simulink model "TractorTrailer6DOF"  (R2023b)
settings: Solver=ode23tb  StartTime=0.0  StopTime=50  MaxStep=1.0  RelTol=1e-1  AbsTol=1e-5
model mask{initialTractorPosition=[0 0 0], initialTractorVelocity=[0 0 0], initialTractorOrientation=[0 0 0], initialTractorRotationRates=[0 0 0], initialTrailerPosition=[0 0 0], initialTrailerVelocity=[0 0 0], initialTrailerOrientation=[0 0 0], initialTrailerRotationRates=[0 0 0]}
  mask prompts: initialTractorPosition "Initial Tractor Position:"; initialTractorVelocity "Initial Tractor Velocity:"; initialTractorOrientation "Initial Tractor Orientation:"; initialTractorRotationRates "Initial Tractor Rotation Rates:"; initialTrailerPosition "Initial Trailer Position:"; initialTrailerVelocity "Initial Trailer Velocity:"; initialTrailerOrientation "Initial Trailer Orientation:"; initialTrailerRotationRates "Initial Trailer Rotation Rates:"
model workspace (MAT data in the model file):
  initialTractorOrientation : Simulink.Parameter (value not decoded)
  initialTractorPosition : Simulink.Parameter (value not decoded)
  initialTractorRotationRates : Simulink.Parameter (value not decoded)
  initialTractorVelocity : Simulink.Parameter (value not decoded)
  initialTrailerOrientation : Simulink.Parameter (value not decoded)
  initialTrailerPosition : Simulink.Parameter (value not decoded)
  initialTrailerRotationRates : Simulink.Parameter (value not decoded)
  initialTrailerVelocity : Simulink.Parameter (value not decoded)
undefined symbols (not defined in the file): hitch, tractor, trailer
libraries: autolibutils x7, sharedtransform x4, vehdynlibtire x4, vehdynlibeom x2, vehdynlibsuspension x2, vehdynlibtirecommon x2, simulink x1
(part 2 of 4)

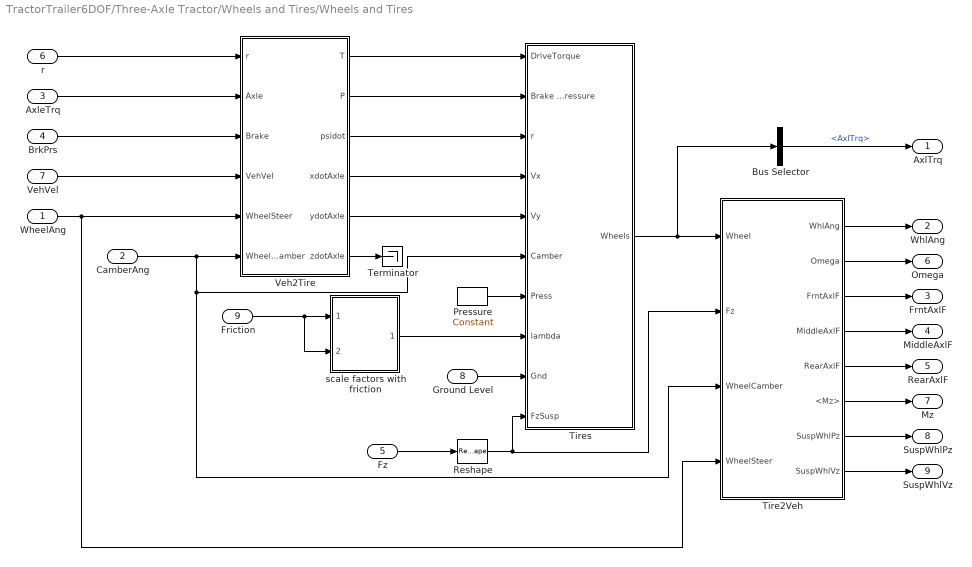
== system TractorTrailer6DOF/Three-Axle Tractor/Wheels and Tires/Wheels and Tires ==
  WheelAng : Inport
  CamberAng : Inport  Port=2  Unit=rad
  AxleTrq : Inport  Port=3
  BrkPrs : Inport  Port=4
  Fz : Inport  Port=5  Unit=N
  r : Inport  Port=6
  VehVel : Inport  Port=7
  Ground Level : Inport  Port=8
  Friction : Inport  Port=9  Unit=1
  Bus Selector : BusSelector  OutputSignals=AxlTrq
  Pressure : vehdynlibtirecommon/Constant  const=220000  numWheels=6
  Reshape : Reshape
  Terminator : Terminator
  Tire2Veh : Subsystem
  Tires : Subsystem  Variant=on  VariantControlMode=label  VariantControl=Variant1  LabelModeActiveChoice=0
  Veh2Tire : Subsystem
  scale factors with friction : Subsystem  mask{numWheels=6}
      mask prompts: numWheels "Number of wheels"
  AxlTrq : Outport
  WhlAng : Outport  Port=2  VectorParamsAs1DForOutWhenUnconnected=off
  FrntAxlF : Outport  Port=3  Unit=N  VectorParamsAs1DForOutWhenUnconnected=off
  MiddleAxlF : Outport  Port=4  Unit=N  VectorParamsAs1DForOutWhenUnconnected=off
  RearAxlF : Outport  Port=5  Unit=N  VectorParamsAs1DForOutWhenUnconnected=off
  Omega : Outport  Port=6  VectorParamsAs1DForOutWhenUnconnected=off
  Mz : Outport  Port=7  Unit=N*m  VectorParamsAs1DForOutWhenUnconnected=off
  SuspWhlPz : Outport  Port=8  VectorParamsAs1DForOutWhenUnconnected=off
  SuspWhlVz : Outport  Port=9  VectorParamsAs1DForOutWhenUnconnected=off
  wires:
  Ground Level/1 -> Tires/9("Gnd ")
  Pressure/1 -> Tires/7("Press ")
  scale factors with friction/1(lambdas) -> Tires/8("lambda ")
  Fz/1 -> Reshape/1
  AxleTrq/1 -> Veh2Tire/2(Axle)
  BrkPrs/1 -> Veh2Tire/3(Brake)
  VehVel/1 -> Veh2Tire/4(VehVel)
  Veh2Tire/1(T) -> Tires/1("DriveTorque ")
  Veh2Tire/2(P) -> Tires/2("Brake Pressure ")
  Veh2Tire/4(xdotAxle) -> Tires/4("Vx ")
  Veh2Tire/5(ydotAxle) -> Tires/5("Vy ")
  Veh2Tire/3(psidot) -> Tires/3("r ")
  Tires/1(" Wheels") -> Bus Selector/1, Tire2Veh/1(Wheel)
  WheelAng/1 -> Veh2Tire/5(WheelSteer), Tire2Veh/4(WheelSteer)
  Tire2Veh/2(Omega) -> Omega/1
  Tire2Veh/3(FrntAxlF) -> FrntAxlF/1
  Tire2Veh/4(MiddleAxlF) -> MiddleAxlF/1
  Tire2Veh/6(<Mz>) -> Mz/1
  Friction/1 -> scale factors with friction/2(lamda_mu_y), scale factors with friction/1(lamda_mu_x)
  r/1 -> Veh2Tire/1(r)
  Veh2Tire/6(zdotAxle) -> Terminator/1
  Tire2Veh/7(SuspWhlPz) -> SuspWhlPz/1
  Tire2Veh/8(SuspWhlVz) -> SuspWhlVz/1
  CamberAng/1 -> Tires/6("Camber "), Tire2Veh/3(WheelCamber), Veh2Tire/6(WheelCamber)
  Tire2Veh/1(WhlAng) -> WhlAng/1
  Tire2Veh/5(RearAxlF) -> RearAxlF/1
  Reshape/1 -> Tires/10("FzSusp "), Tire2Veh/2(Fz)
  Bus Selector/1 -> AxlTrq/1  "<AxlTrq>"

== system TractorTrailer6DOF/Three-Axle Tractor/Wheels and Tires/z forces per tire ==
  FzIn : Inport
  Demux : Demux  Outputs=6
  Gain10 : Gain  Gain=1/tractor.NumberOfWheelsPerMiddleAxle
  Gain11 : Gain  Gain=1/tractor.NumberOfWheelsPerMiddleAxle
  Gain12 : Gain  Gain=1/tractor.NumberOfWheelsPerRearAxle
  Gain13 : Gain  Gain=1/tractor.NumberOfWheelsPerRearAxle
  Gain14 : Gain  Gain=2
  Gain8 : Gain  Gain=1/tractor.NumberOfWheelsPerFrontAxle
  Gain9 : Gain  Gain=1/tractor.NumberOfWheelsPerFrontAxle
  Mux1 : Mux  Inputs=6
  FzTire : Outport
  wires:
  Gain12/1 -> Mux1/5
  Gain13/1 -> Mux1/6
  Gain11/1 -> Mux1/4
  Demux/2 -> Gain9/1
  Gain14/1 -> FzTire/1
  Gain8/1 -> Mux1/1
  Mux1/1 -> Gain14/1
  Gain10/1 -> Mux1/3
  Demux/6 -> Gain13/1
  Gain9/1 -> Mux1/2
  Demux/3 -> Gain10/1
  Demux/4 -> Gain11/1
  Demux/1 -> Gain8/1
  Demux/5 -> Gain12/1
  FzIn/1 -> Demux/1

== system TractorTrailer6DOF/Three-Axle Trailer/Trailer Suspension/Steer Rate Adapter ==
  Veh : Inport
  Add : Sum
  Bus Selector3 : BusSelector  OutputSignals=BdyFrm.Cg.AngVel.r
  Constant : Constant  Value=zeros(1,6)
  Matrix Concatenate : Concatenate  NumInputs=3  Mode=Multidimensional array
  Matrix Concatenate1 : Concatenate  NumInputs=3  Mode=Multidimensional array
  Mux : Mux  Inputs=6
  Reshape2 : Reshape  OutputDimensionality=Row vector (2-D)
  Reshape3 : Reshape  OutputDimensionality=Row vector (2-D)
  Reshape4 : Reshape  OutputDimensionality=Row vector (2-D)
  SteerRates : Constant  Value=zeros(1,6)
  AngVel : Outport  VectorParamsAs1DForOutWhenUnconnected=off
  wires:
  Add/1 -> AngVel/1  "AngVel"
  Veh/1 -> Bus Selector3/1
  Matrix Concatenate1/1 -> Add/1
  Reshape3/1 -> Matrix Concatenate/1, Matrix Concatenate/2
  Reshape4/1 -> Matrix Concatenate/3
  SteerRates/1 -> Reshape2/1
  Matrix Concatenate/1 -> Add/2
  Bus Selector3/1 -> Mux/1, Mux/3, Mux/6, Mux/5, Mux/4, Mux/2  "<r>"
  Mux/1 -> Reshape4/1
  Constant/1 -> Reshape3/1
  Reshape2/1 -> Matrix Concatenate1/2, Matrix Concatenate1/3, Matrix Concatenate1/1

== system TractorTrailer6DOF/Three-Axle Trailer/Trailer Suspension/Steering Adapter ==
  Steer : Inport
  Reshape1 : Reshape  OutputDimensionality=Row vector (2-D)
  StrgAng : Outport  VectorParamsAs1DForOutWhenUnconnected=off
  wires:
  Steer/1 -> Reshape1/1
  Reshape1/1 -> StrgAng/1

== system TractorTrailer6DOF/Three-Axle Trailer/Trailer Suspension/Vehicle Adapter ==
  Veh : Inport
  Bus Creator3 : BusCreator  Inputs=2
  Bus Selector1 : BusSelector  OutputSignals=InertFrm.FrntAxl.Lft.Disp.X,InertFrm.FrntAxl.Lft.Disp.Y,InertFrm.FrntAxl.Lft.Disp.Z,InertFrm.FrntAxl.Rght.Disp.X,InertFrm.FrntAxl.Rght.Disp.Y,InertFrm.FrntAxl.Rght.Disp.Z,InertFrm.MidlAxl.Lft.Disp.X,InertFrm.MidlAxl.Lft.Disp.Y,InertFrm.MidlAxl.Lft.Disp.Z,InertFrm.MidlAxl.Rght.Disp.X,InertFrm.MidlAxl.Rght.Disp.Y,InertFrm.MidlAxl.Rght.Disp.Z,InertFrm.RearAxl.Lft.Disp.X,InertFrm.RearAxl.Lft.Disp.Y,InertFrm.RearAxl.Lft.Disp.Z,InertFrm.RearAxl.Rght.Disp.X,InertFrm.RearAxl.Rght.Disp.Y,InertFrm.RearAxl.Rght.Disp.Z
  Bus Selector2 : BusSelector  OutputSignals=BdyFrm.FrntAxl.Lft.Vel.xdot,BdyFrm.FrntAxl.Lft.Vel.ydot,BdyFrm.FrntAxl.Lft.Vel.zdot,BdyFrm.FrntAxl.Rght.Vel.xdot,BdyFrm.FrntAxl.Rght.Vel.ydot,BdyFrm.FrntAxl.Rght.Vel.zdot,BdyFrm.MidlAxl.Lft.Vel.xdot,BdyFrm.MidlAxl.Lft.Vel.ydot,BdyFrm.MidlAxl.Lft.Vel.zdot,BdyFrm.MidlAxl.Rght.Vel.xdot,BdyFrm.MidlAxl.Rght.Vel.ydot,BdyFrm.MidlAxl.Rght.Vel.zdot,BdyFrm.RearAxl.Lft.Vel.xdot,BdyFrm.RearAxl.Lft.Vel.ydot,BdyFrm.RearAxl.Lft.Vel.zdot,BdyFrm.RearAxl.Rght.Vel.xdot,BdyFrm.RearAxl.Rght.Vel.ydot,BdyFrm.RearAxl.Rght.Vel.zdot
  Bus Selector3 : BusSelector  OutputSignals=InertFrm.FrntAxl.Lft.Vel.Xdot,InertFrm.FrntAxl.Lft.Vel.Ydot,InertFrm.FrntAxl.Lft.Vel.Zdot,InertFrm.FrntAxl.Rght.Vel.Xdot,InertFrm.FrntAxl.Rght.Vel.Ydot,InertFrm.FrntAxl.Rght.Vel.Zdot,InertFrm.MidlAxl.Lft.Vel.Xdot,InertFrm.MidlAxl.Lft.Vel.Ydot,InertFrm.MidlAxl.Lft.Vel.Zdot,InertFrm.MidlAxl.Rght.Vel.Xdot,InertFrm.MidlAxl.Rght.Vel.Ydot,InertFrm.MidlAxl.Rght.Vel.Zdot,InertFrm.RearAxl.Lft.Vel.Xdot,InertFrm.RearAxl.Lft.Vel.Ydot,InertFrm.RearAxl.Lft.Vel.Zdot,InertFrm.RearAxl.Rght.Vel.Xdot,InertFrm.RearAxl.Rght.Vel.Ydot,InertFrm.RearAxl.Rght.Vel.Zdot
  Inertial Frame CG to Axle Offset : Constant  Value=[zeros(2,6);trailer.HeightCG*ones(1,6)]
  Mux1 : Mux  Inputs=18
  Mux2 : Mux  Inputs=18
  Mux3 : Mux  Inputs=18
  Reshape : Reshape  OutputDimensionality=Customize  OutputDimensions=[3,6]
  Reshape1 : Reshape  OutputDimensionality=Customize  OutputDimensions=[3,6]
  Reshape2 : Reshape  OutputDimensionality=Customize  OutputDimensions=[3,6]
  Sum : Sum  Inputs=|+-
  VehVBody : Outport  VectorParamsAs1DForOutWhenUnconnected=off
  VehSusp : Outport  Port=2  VectorParamsAs1DForOutWhenUnconnected=off
  wires:
  Bus Selector2/18 -> Mux1/18  "<zdot>"
  Bus Selector2/17 -> Mux1/17  "<ydot>"
  Bus Selector2/16 -> Mux1/16  "<xdot>"
  Bus Selector2/15 -> Mux1/15  "<zdot>"
  Bus Selector2/14 -> Mux1/14  "<ydot>"
  Bus Selector2/13 -> Mux1/13  "<xdot>"
  Bus Selector2/12 -> Mux1/12  "<zdot>"
  Bus Selector2/11 -> Mux1/11  "<ydot>"
  Bus Selector2/10 -> Mux1/10  "<xdot>"
  Bus Selector2/9 -> Mux1/9  "<zdot>"
  Bus Selector2/8 -> Mux1/8  "<ydot>"
  Bus Selector2/7 -> Mux1/7  "<xdot>"
  Bus Selector2/6 -> Mux1/6  "<zdot>"
  Bus Selector2/5 -> Mux1/5  "<ydot>"
  Bus Selector2/4 -> Mux1/4  "<xdot>"
  Bus Selector2/3 -> Mux1/3  "<zdot>"
  Bus Selector2/2 -> Mux1/2  "<ydot>"
  Bus Selector2/1 -> Mux1/1  "<xdot>"
  Bus Selector1/18 -> Mux2/18  "<Z>"
  Bus Selector1/17 -> Mux2/17  "<Y>"
  Bus Selector1/16 -> Mux2/16  "<X>"
  Bus Selector1/15 -> Mux2/15  "<Z>"
  Bus Selector1/14 -> Mux2/14  "<Y>"
  Bus Selector1/13 -> Mux2/13  "<X>"
  Bus Selector1/12 -> Mux2/12  "<Z>"
  Bus Selector1/11 -> Mux2/11  "<Y>"
  Bus Selector1/10 -> Mux2/10  "<X>"
  Bus Selector1/9 -> Mux2/9  "<Z>"
  Bus Selector1/8 -> Mux2/8  "<Y>"
  Bus Selector1/7 -> Mux2/7  "<X>"
  Bus Selector1/6 -> Mux2/6  "<Z>"
  Bus Selector1/5 -> Mux2/5  "<Y>"
  Bus Selector1/4 -> Mux2/4  "<X>"
  Bus Selector1/3 -> Mux2/3  "<Z>"
  Bus Selector1/2 -> Mux2/2  "<Y>"
  Bus Selector1/1 -> Mux2/1  "<X>"
  Sum/1 -> Bus Creator3/1  "P"
  Inertial Frame CG to Axle Offset/1 -> Sum/2
  Mux2/1 -> Reshape/1
  Mux1/1 -> Reshape2/1
  Reshape/1 -> Sum/1
  Bus Creator3/1 -> VehSusp/1  "Veh"
  Reshape2/1 -> VehVBody/1  "V"
  Veh/1 -> Bus Selector1/1, Bus Selector2/1, Bus Selector3/1
  Reshape1/1 -> Bus Creator3/2  "V"
  Mux3/1 -> Reshape1/1
  Bus Selector3/1 -> Mux3/1  "<Xdot>"
  Bus Selector3/2 -> Mux3/2  "<Ydot>"
  Bus Selector3/3 -> Mux3/3  "<Zdot>"
  Bus Selector3/4 -> Mux3/4  "<Xdot>"
  Bus Selector3/5 -> Mux3/5  "<Ydot>"
  Bus Selector3/6 -> Mux3/6  "<Zdot>"
  Bus Selector3/7 -> Mux3/7  "<Xdot>"
  Bus Selector3/8 -> Mux3/8  "<Ydot>"
  Bus Selector3/9 -> Mux3/9  "<Zdot>"
  Bus Selector3/10 -> Mux3/10  "<Xdot>"
  Bus Selector3/11 -> Mux3/11  "<Ydot>"
  Bus Selector3/12 -> Mux3/12  "<Zdot>"
  Bus Selector3/13 -> Mux3/13  "<Xdot>"
  Bus Selector3/14 -> Mux3/14  "<Ydot>"
  Bus Selector3/15 -> Mux3/15  "<Zdot>"
  Bus Selector3/16 -> Mux3/16  "<Xdot>"
  Bus Selector3/17 -> Mux3/17  "<Ydot>"
  Bus Selector3/18 -> Mux3/18  "<Zdot>"

== system TractorTrailer6DOF/Three-Axle Trailer/Trailer Suspension/Wheel  Adapter ==
  Wheels : Inport
  Bus Selector : BusSelector  OutputSignals=TireFrame.Fx,TireFrame.Fy
  Bus Selector1 : BusSelector  OutputSignals=TireFrame.Re
  Bus Selector2 : BusSelector  OutputSignals=TireFrame.Mx,TireFrame.My,TireFrame.Mz
  Bus Selector3 : BusSelector  OutputSignals=TireFrame.z,TireFrame.zdot
  Matrix Concatenate : Concatenate  NumInputs=3  Mode=Multidimensional array
  Reshape{,1..7} (8 alike) : Reshape  OutputDimensionality=Row vector (2-D)
  WhlFx : Outport  VectorParamsAs1DForOutWhenUnconnected=off
  WhlFy : Outport  Port=2  VectorParamsAs1DForOutWhenUnconnected=off
  z : Outport  Port=3  VectorParamsAs1DForOutWhenUnconnected=off
  zdot : Outport  Port=4  VectorParamsAs1DForOutWhenUnconnected=off
  M : Outport  Port=5  VectorParamsAs1DForOutWhenUnconnected=off
  Re : Outport  Port=6  VectorParamsAs1DForOutWhenUnconnected=off
  wires:
  Reshape/1 -> z/1  "z"
  Matrix Concatenate/1 -> M/1  "M"
  Reshape5/1 -> Matrix Concatenate/3
  Reshape4/1 -> Matrix Concatenate/2
  Reshape3/1 -> Matrix Concatenate/1
  Bus Selector2/3 -> Reshape5/1  "<Mz>"
  Bus Selector2/2 -> Reshape4/1  "<My>"
  Bus Selector2/1 -> Reshape3/1  "<Mx>"
  Reshape1/1 -> Re/1  "Re"
  Bus Selector1/1 -> Reshape1/1  "<Re>"
  Reshape2/1 -> zdot/1  "zdot"
  Bus Selector3/2 -> Reshape2/1  "<zdot>"
  Wheels/1 -> Bus Selector/1, Bus Selector3/1, Bus Selector2/1, Bus Selector1/1
  Bus Selector3/1 -> Reshape/1  "<z>"
  Bus Selector/2 -> Reshape7/1  "<Fy>"
  Bus Selector/1 -> Reshape6/1  "<Fx>"
  Reshape6/1 -> WhlFx/1
  Reshape7/1 -> WhlFy/1

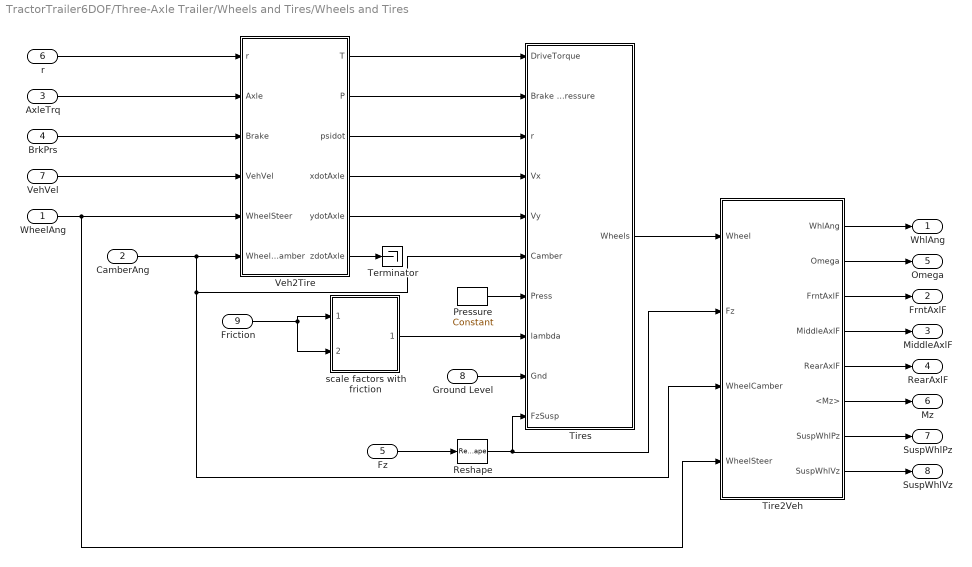
== system TractorTrailer6DOF/Three-Axle Trailer/Wheels and Tires/Wheels and Tires ==
  WheelAng : Inport
  CamberAng : Inport  Port=2  Unit=rad
  AxleTrq : Inport  Port=3
  BrkPrs : Inport  Port=4
  Fz : Inport  Port=5  Unit=N
  r : Inport  Port=6
  VehVel : Inport  Port=7
  Ground Level : Inport  Port=8
  Friction : Inport  Port=9  Unit=1
  Pressure : vehdynlibtirecommon/Constant  const=220000  numWheels=6
  Reshape : Reshape
  Terminator : Terminator
  Tire2Veh : Subsystem
  Tires : Subsystem  Variant=on  VariantControlMode=label  VariantControl=Variant1  LabelModeActiveChoice=0
  Veh2Tire : Subsystem
  scale factors with friction : Subsystem  mask{numWheels=6}
      mask prompts: numWheels "Number of wheels"
  WhlAng : Outport  VectorParamsAs1DForOutWhenUnconnected=off
  FrntAxlF : Outport  Port=2  Unit=N  VectorParamsAs1DForOutWhenUnconnected=off
  MiddleAxlF : Outport  Port=3  Unit=N  VectorParamsAs1DForOutWhenUnconnected=off
  RearAxlF : Outport  Port=4  Unit=N  VectorParamsAs1DForOutWhenUnconnected=off
  Omega : Outport  Port=5  VectorParamsAs1DForOutWhenUnconnected=off
  Mz : Outport  Port=6  Unit=N*m  VectorParamsAs1DForOutWhenUnconnected=off
  SuspWhlPz : Outport  Port=7  VectorParamsAs1DForOutWhenUnconnected=off
  SuspWhlVz : Outport  Port=8  VectorParamsAs1DForOutWhenUnconnected=off
  wires:
  Reshape/1 -> Tire2Veh/2(Fz), Tires/10("FzSusp ")
  Tire2Veh/5(RearAxlF) -> RearAxlF/1
  Tire2Veh/1(WhlAng) -> WhlAng/1
  CamberAng/1 -> Veh2Tire/6(WheelCamber), Tire2Veh/3(WheelCamber), Tires/6("Camber ")
  Tire2Veh/8(SuspWhlVz) -> SuspWhlVz/1
  Tire2Veh/7(SuspWhlPz) -> SuspWhlPz/1
  Veh2Tire/6(zdotAxle) -> Terminator/1
  r/1 -> Veh2Tire/1(r)
  Friction/1 -> scale factors with friction/2(lamda_mu_y), scale factors with friction/1(lamda_mu_x)
  Tire2Veh/6(<Mz>) -> Mz/1
  Tire2Veh/4(MiddleAxlF) -> MiddleAxlF/1
  Tire2Veh/3(FrntAxlF) -> FrntAxlF/1
  Tire2Veh/2(Omega) -> Omega/1
  WheelAng/1 -> Tire2Veh/4(WheelSteer), Veh2Tire/5(WheelSteer)
  Tires/1(" Wheels") -> Tire2Veh/1(Wheel)
  Veh2Tire/3(psidot) -> Tires/3("r ")
  Veh2Tire/5(ydotAxle) -> Tires/5("Vy ")
  Veh2Tire/4(xdotAxle) -> Tires/4("Vx ")
  Veh2Tire/2(P) -> Tires/2("Brake Pressure ")
  Veh2Tire/1(T) -> Tires/1("DriveTorque ")
  VehVel/1 -> Veh2Tire/4(VehVel)
  BrkPrs/1 -> Veh2Tire/3(Brake)
  AxleTrq/1 -> Veh2Tire/2(Axle)
  Fz/1 -> Reshape/1
  scale factors with friction/1(lambdas) -> Tires/8("lambda ")
  Pressure/1 -> Tires/7("Press ")
  Ground Level/1 -> Tires/9("Gnd ")

== system TractorTrailer6DOF/Three-Axle Tractor/Subsystem1/Driveline/AWD ==
  TPowertrain : Inport
  Gear : Inport  Port=2
  AWD : Gain  Gain=[1;1;1;1;1;1]./2
  Add : Sum
  Constant : Constant
  Constant1 : Constant  Value=zeros(6,1)
  Multiport Switch : MultiPortSwitch  DataPortOrder=Zero-based contiguous  zeroidx=on  SaturateOnIntegerOverflow=off  InputSameDT=off
  Unary Minus : UnaryMinus
  TAxles : Outport  VectorParamsAs1DForOutWhenUnconnected=off
  wires:
  Unary Minus/1 -> Multiport Switch/2
  Gear/1 -> Add/1
  Constant/1 -> Add/2
  AWD/1 -> Multiport Switch/4, Unary Minus/1
  Constant1/1 -> Multiport Switch/3
  Add/1 -> Multiport Switch/1
  Multiport Switch/1 -> TAxles/1
  TPowertrain/1 -> AWD/1

== system TractorTrailer6DOF/Three-Axle Tractor/Subsystem1/Driveline/FWD ==
  TPowertrain : Inport
  Gear : Inport  Port=2
  Add : Sum
  Constant : Constant
  Constant1 : Constant  Value=zeros(6,1)
  FWD : Gain  Gain=[1;1;0;0;0;0]
  Multiport Switch : MultiPortSwitch  DataPortOrder=Zero-based contiguous  zeroidx=on  SaturateOnIntegerOverflow=off  InputSameDT=off
  Unary Minus : UnaryMinus
  TAxles : Outport  VectorParamsAs1DForOutWhenUnconnected=off
  wires:
  Unary Minus/1 -> Multiport Switch/2
  Gear/1 -> Add/1
  Constant/1 -> Add/2
  FWD/1 -> Multiport Switch/4, Unary Minus/1
  Constant1/1 -> Multiport Switch/3
  Add/1 -> Multiport Switch/1
  Multiport Switch/1 -> TAxles/1
  TPowertrain/1 -> FWD/1

== system TractorTrailer6DOF/Three-Axle Tractor/Subsystem1/Driveline/RWD ==
  TPowertrain : Inport
  Gear : Inport  Port=2
  Add : Sum
  Constant : Constant
  Constant1 : Constant  Value=zeros(6,1)
  Constant2 : Constant  Value=0
  Multiport Switch : MultiPortSwitch  DataPortOrder=Zero-based contiguous  zeroidx=on  SaturateOnIntegerOverflow=off  InputSameDT=off
  Mux : Mux  Inputs=6
  Unary Minus : UnaryMinus
  TAxles : Outport  VectorParamsAs1DForOutWhenUnconnected=off
  wires:
  Constant1/1 -> Multiport Switch/3
  Add/1 -> Multiport Switch/1
  Constant/1 -> Add/2
  Gear/1 -> Add/1
  Multiport Switch/1 -> TAxles/1
  Unary Minus/1 -> Multiport Switch/2
  Mux/1 -> Multiport Switch/4, Unary Minus/1
  TPowertrain/1 -> Mux/6, Mux/5
  Constant2/1 -> Mux/4, Mux/3, Mux/2, Mux/1

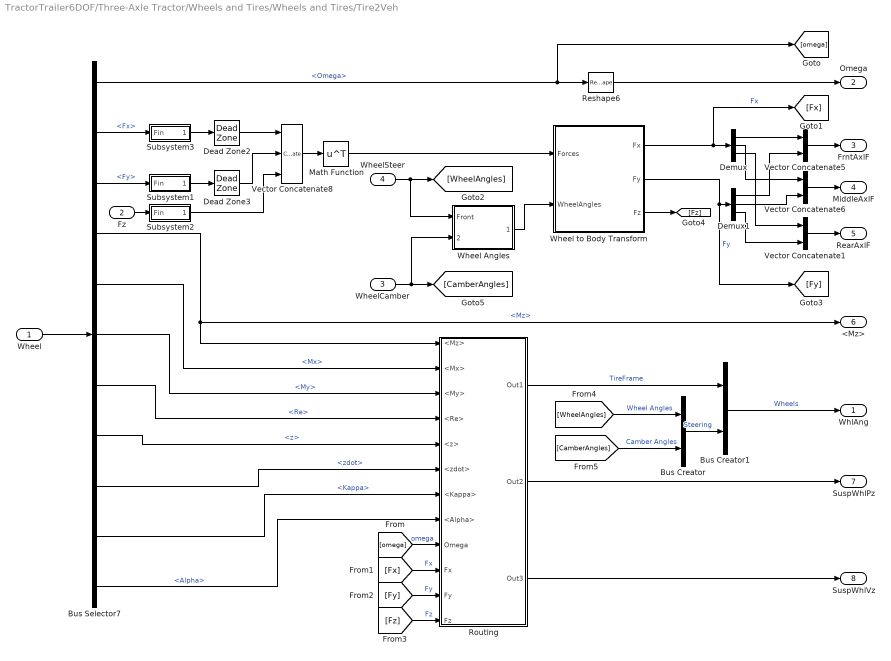
== system TractorTrailer6DOF/Three-Axle Tractor/Wheels and Tires/Wheels and Tires/Tire2Veh ==
  Wheel : Inport
  Fz : Inport  Port=2
  WheelCamber : Inport  Port=3
  WheelSteer : Inport  Port=4
  Bus Creator : BusCreator  Inputs=2
  Bus Creator1 : BusCreator  Inputs=2
  Bus Selector7 : BusSelector  OutputSignals=Omega,Fx,Fy,Mz,Mx,My,Re,z,zdot,Kappa,Alpha
  Dead Zone2 : DeadZone  LowerValue=-5  UpperValue=5  ZeroCross=off
  Dead Zone3 : DeadZone  LowerValue=-10  UpperValue=10  ZeroCross=off
  Demux : Demux  Outputs=[2,2,2]
  Demux1 : Demux  Outputs=[2,2,2]
  Math Function : Math  Operator=transpose  SignedPower=on
  Reshape6 : Reshape  OutputDimensionality=Customize  OutputDimensions=[3,2]
  Routing : Subsystem
  Subsystem1 : Subsystem
  Subsystem2 : Subsystem
  Subsystem3 : Subsystem
  Vector Concatenate1 : Concatenate  Mode=Multidimensional array  ConcatenateDimension=2
  Vector Concatenate5 : Concatenate  Mode=Multidimensional array  ConcatenateDimension=2
  Vector Concatenate6 : Concatenate  Mode=Multidimensional array  ConcatenateDimension=2
  Vector Concatenate8 : Concatenate  NumInputs=3  Mode=Multidimensional array  ConcatenateDimension=2
  Wheel Angles : Subsystem
  Wheel to Body Transform : Subsystem
  WhlAng : Outport  VectorParamsAs1DForOutWhenUnconnected=off
  Omega : Outport  Port=2  VectorParamsAs1DForOutWhenUnconnected=off
  FrntAxlF : Outport  Port=3  VectorParamsAs1DForOutWhenUnconnected=off
  MiddleAxlF : Outport  Port=4  VectorParamsAs1DForOutWhenUnconnected=off
  RearAxlF : Outport  Port=5  VectorParamsAs1DForOutWhenUnconnected=off
  <Mz> : Outport  Port=6  VectorParamsAs1DForOutWhenUnconnected=off
  SuspWhlPz : Outport  Port=7  VectorParamsAs1DForOutWhenUnconnected=off
  SuspWhlVz : Outport  Port=8  VectorParamsAs1DForOutWhenUnconnected=off
  wires:
  Fz/1 -> Subsystem2/1(Fin)
  Vector Concatenate6/1 -> MiddleAxlF/1
  Vector Concatenate8/1 -> Math Function/1
  Demux/2 -> Vector Concatenate6/1
  Demux1/2 -> Vector Concatenate6/2
  Demux/1 -> Vector Concatenate5/1
  Math Function/1 -> Wheel to Body Transform/1(Forces)
  Dead Zone3/1 -> Vector Concatenate8/2
  Bus Selector7/2 -> Subsystem3/1(Fin)  "<Fx>"
  Dead Zone2/1 -> Vector Concatenate8/1
  Wheel to Body Transform/1(Fx) -> [Fx], Demux/1  "Fx"
  Vector Concatenate5/1 -> FrntAxlF/1
  Wheel/1 -> Bus Selector7/1
  Reshape6/1 -> Omega/1
  Demux1/1 -> Vector Concatenate5/2
  Wheel to Body Transform/2(Fy) -> Demux1/1, [Fy]  "Fy"
  Wheel Angles/1(Vehicle) -> Wheel to Body Transform/2(WheelAngles)
  Bus Selector7/1 -> [omega], Reshape6/1  "<Omega>"
  WheelSteer/1 -> Wheel Angles/1(Front), [WheelAngles]
  Bus Selector7/4 -> <Mz>/1, Routing/1(<Mz>)  "<Mz>"
  Wheel to Body Transform/3(Fz) -> [Fz]
  WheelCamber/1 -> Wheel Angles/2(Camber), [CamberAngles]
  Bus Selector7/3 -> Subsystem1/1(Fin)  "<Fy>"
  Bus Selector7/5 -> Routing/2(<Mx>)  "<Mx>"
  Bus Selector7/6 -> Routing/3(<My>)  "<My>"
  Bus Selector7/7 -> Routing/4(<Re>)  "<Re>"
  [omega] -> Routing/9(Omega)  "omega"
  [Fx] -> Routing/10(Fx)  "Fx"
  Bus Selector7/8 -> Routing/5(<z>)  "<z>"
  [Fy] -> Routing/11(Fy)  "Fy"
  [Fz] -> Routing/12(Fz)  "Fz"
  Bus Selector7/9 -> Routing/6(<zdot>)  "<zdot>"
  Bus Selector7/10 -> Routing/7(<Kappa>)  "<Kappa>"
  Routing/2(Out2) -> SuspWhlPz/1
  Routing/3(Out3) -> SuspWhlVz/1
  [WheelAngles] -> Bus Creator/1  "Wheel Angles"
  Bus Creator1/1 -> WhlAng/1  "Wheels"
  Routing/1(Out1) -> Bus Creator1/1  "TireFrame"
  [CamberAngles] -> Bus Creator/2  "Camber Angles"
  Bus Creator/1 -> Bus Creator1/2  "Steering"
  Bus Selector7/11 -> Routing/8(<Alpha>)  "<Alpha>"
  Vector Concatenate1/1 -> RearAxlF/1
  Demux/3 -> Vector Concatenate1/1
  Demux1/3 -> Vector Concatenate1/2
  Subsystem2/1(Fout) -> Vector Concatenate8/3
  Subsystem1/1(Fout) -> Dead Zone3/1
  Subsystem3/1(Fout) -> Dead Zone2/1

== system TractorTrailer6DOF/Three-Axle Tractor/Wheels and Tires/Wheels and Tires/Tires ==
  "DriveTorque " : Inport
  "Brake Pressure " : Inport  Port=2
  "r " : Inport  Port=3
  "Vx " : Inport  Port=4
  "Vy " : Inport  Port=5
  "Camber " : Inport  Port=6
  "Press " : Inport  Port=7
  "lambda " : Inport  Port=8
  "Gnd " : Inport  Port=9
  "FzSusp " : Inport  Port=10
  Fiala Tires : Subsystem  VariantControl=1
  MF Tires : Subsystem  VariantControl=0
  " Wheels" : Outport  VectorParamsAs1DForOutWhenUnconnected=off

== system TractorTrailer6DOF/Three-Axle Tractor/Wheels and Tires/Wheels and Tires/Veh2Tire ==
  r : Inport
  Axle : Inport  Port=2
  Brake : Inport  Port=3
  VehVel : Inport  Port=4
  WheelSteer : Inport  Port=5
  WheelCamber : Inport  Port=6
  Demux4 : Demux  Outputs=6
  Gain4 : Gain  Gain=[1;-1;1;-1;1;-1]*0+1
  Mux1 : Mux  Inputs=6
  Reshape3 : Reshape
  Reshape4 : Reshape
  Unary Minus : UnaryMinus
  Wheel Angles : Subsystem
  Wheel to Body Transform : Subsystem
  T : Outport  Unit=N*m  VectorParamsAs1DForOutWhenUnconnected=off
  P : Outport  Port=2  Unit=Pa  VectorParamsAs1DForOutWhenUnconnected=off
  psidot : Outport  Port=3  Unit=rad/s  VectorParamsAs1DForOutWhenUnconnected=off
  xdotAxle : Outport  Port=4  Unit=m/s  VectorParamsAs1DForOutWhenUnconnected=off
  ydotAxle : Outport  Port=5  Unit=m/s  VectorParamsAs1DForOutWhenUnconnected=off
  zdotAxle : Outport  Port=6  Unit=m/s  VectorParamsAs1DForOutWhenUnconnected=off
  wires:
  Demux4/1 -> Mux1/1
  Brake/1 -> Reshape3/1
  Demux4/4 -> Mux1/4
  Axle/1 -> Reshape4/1
  Wheel to Body Transform/1(xdotWheel) -> xdotAxle/1  "Vx"
  Demux4/2 -> Mux1/2
  Wheel to Body Transform/2(ydotWheel) -> ydotAxle/1  "Vy"
  WheelSteer/1 -> Wheel Angles/1(steer)
  Mux1/1 -> P/1
  r/1 -> Unary Minus/1
  Demux4/3 -> Mux1/3
  Reshape3/1 -> Demux4/1
  Gain4/1 -> T/1
  Reshape4/1 -> Gain4/1
  VehVel/1 -> Wheel to Body Transform/1(VelVeh)
  Wheel to Body Transform/3(zdotWheel) -> zdotAxle/1  "Vz"
  WheelCamber/1 -> Wheel Angles/2(camber)
  Unary Minus/1 -> psidot/1
  Wheel Angles/1(Vehicle) -> Wheel to Body Transform/2(WheelAngles)
  Demux4/5 -> Mux1/5
  Demux4/6 -> Mux1/6

== system TractorTrailer6DOF/Three-Axle Tractor/Wheels and Tires/Wheels and Tires/scale factors with friction ==
  lamda_mu_x : Inport
  lamda_mu_y : Inport  Port=2
  0 : Constant  Value=[zeros(1,numWheels)]  VectorParams1D=off
  Reshape : Reshape  OutputDimensionality=Row vector (2-D)  OutputDimensions=[1,numWheels]
  Reshape1 : Reshape  OutputDimensionality=Row vector (2-D)  OutputDimensions=[1,numWheels]
  Signal Specification3 : SignalSpecification  Unit=1
  Vector Concatenate : Concatenate  NumInputs=5  Mode=Multidimensional array
  ones : Constant  Value=[ones(23,numWheels)]  VectorParams1D=off
  ones2 : Constant  Value=ones(1,numWheels)  VectorParams1D=off
  lambdas : Outport  Unit=1  VectorParamsAs1DForOutWhenUnconnected=off
  wires:
  lamda_mu_y/1 -> Reshape1/1
  lamda_mu_x/1 -> Reshape/1
  ones2/1 -> Vector Concatenate/1  "lambda_Fz0"
  Vector Concatenate/1 -> Signal Specification3/1
  ones/1 -> Vector Concatenate/5
  0/1 -> Vector Concatenate/4  "lamda_mu_V"
  Reshape1/1 -> Vector Concatenate/3
  Reshape/1 -> Vector Concatenate/2
  Signal Specification3/1 -> lambdas/1

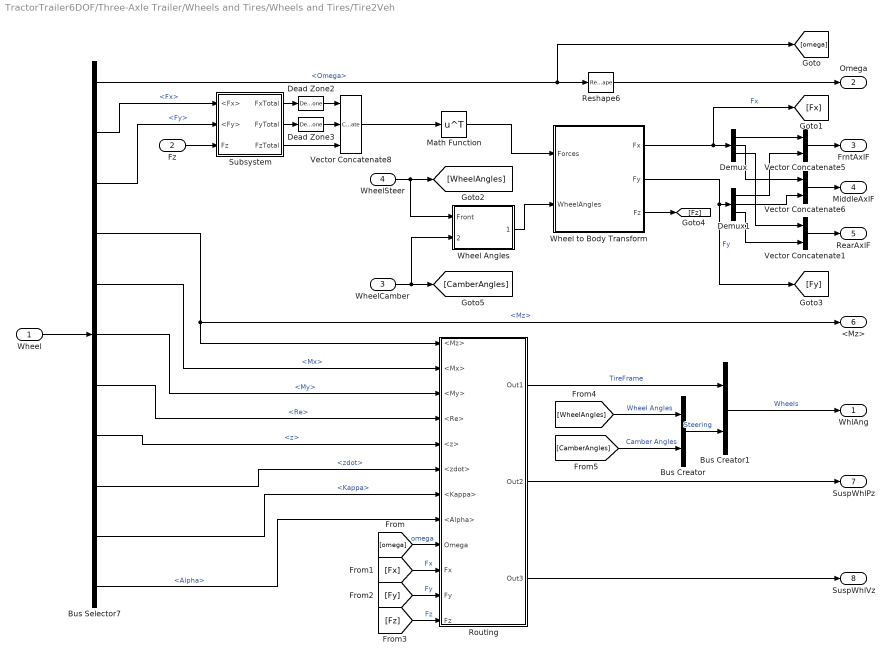
== system TractorTrailer6DOF/Three-Axle Trailer/Wheels and Tires/Wheels and Tires/Tire2Veh ==
  Wheel : Inport
  Fz : Inport  Port=2
  WheelCamber : Inport  Port=3
  WheelSteer : Inport  Port=4
  Bus Creator : BusCreator  Inputs=2
  Bus Creator1 : BusCreator  Inputs=2
  Bus Selector7 : BusSelector  OutputSignals=Omega,Fx,Fy,Mz,Mx,My,Re,z,zdot,Kappa,Alpha
  Dead Zone2 : DeadZone  LowerValue=-5  UpperValue=5  ZeroCross=off
  Dead Zone3 : DeadZone  LowerValue=-10  UpperValue=10  ZeroCross=off
  Demux : Demux  Outputs=[2,2,2]
  Demux1 : Demux  Outputs=[2,2,2]
  Math Function : Math  Operator=transpose  SignedPower=on
  Reshape6 : Reshape  OutputDimensionality=Customize  OutputDimensions=[3,2]
  Routing : Subsystem
  Subsystem : Subsystem
  Vector Concatenate1 : Concatenate  Mode=Multidimensional array  ConcatenateDimension=2
  Vector Concatenate5 : Concatenate  Mode=Multidimensional array  ConcatenateDimension=2
  Vector Concatenate6 : Concatenate  Mode=Multidimensional array  ConcatenateDimension=2
  Vector Concatenate8 : Concatenate  NumInputs=3  Mode=Multidimensional array  ConcatenateDimension=2
  Wheel Angles : Subsystem
  Wheel to Body Transform : Subsystem
  WhlAng : Outport  VectorParamsAs1DForOutWhenUnconnected=off
  Omega : Outport  Port=2  VectorParamsAs1DForOutWhenUnconnected=off
  FrntAxlF : Outport  Port=3  VectorParamsAs1DForOutWhenUnconnected=off
  MiddleAxlF : Outport  Port=4  VectorParamsAs1DForOutWhenUnconnected=off
  RearAxlF : Outport  Port=5  VectorParamsAs1DForOutWhenUnconnected=off
  <Mz> : Outport  Port=6  VectorParamsAs1DForOutWhenUnconnected=off
  SuspWhlPz : Outport  Port=7  VectorParamsAs1DForOutWhenUnconnected=off
  SuspWhlVz : Outport  Port=8  VectorParamsAs1DForOutWhenUnconnected=off
  wires:
  Demux1/3 -> Vector Concatenate1/2
  Demux/3 -> Vector Concatenate1/1
  Vector Concatenate1/1 -> RearAxlF/1
  Bus Selector7/11 -> Routing/8(<Alpha>)  "<Alpha>"
  Bus Creator/1 -> Bus Creator1/2  "Steering"
  [CamberAngles] -> Bus Creator/2  "Camber Angles"
  Routing/1(Out1) -> Bus Creator1/1  "TireFrame"
  Bus Creator1/1 -> WhlAng/1  "Wheels"
  [WheelAngles] -> Bus Creator/1  "Wheel Angles"
  Routing/3(Out3) -> SuspWhlVz/1
  Routing/2(Out2) -> SuspWhlPz/1
  Bus Selector7/10 -> Routing/7(<Kappa>)  "<Kappa>"
  Bus Selector7/9 -> Routing/6(<zdot>)  "<zdot>"
  [Fz] -> Routing/12(Fz)  "Fz"
  [Fy] -> Routing/11(Fy)  "Fy"
  Bus Selector7/8 -> Routing/5(<z>)  "<z>"
  [Fx] -> Routing/10(Fx)  "Fx"
  [omega] -> Routing/9(Omega)  "omega"
  Bus Selector7/7 -> Routing/4(<Re>)  "<Re>"
  Bus Selector7/6 -> Routing/3(<My>)  "<My>"
  Bus Selector7/5 -> Routing/2(<Mx>)  "<Mx>"
  WheelCamber/1 -> [CamberAngles], Wheel Angles/2(Camber)
  Wheel to Body Transform/3(Fz) -> [Fz]
  Bus Selector7/4 -> Routing/1(<Mz>), <Mz>/1  "<Mz>"
  WheelSteer/1 -> [WheelAngles], Wheel Angles/1(Front)
  Bus Selector7/1 -> Reshape6/1, [omega]  "<Omega>"
  Wheel Angles/1(Vehicle) -> Wheel to Body Transform/2(WheelAngles)
  Wheel to Body Transform/2(Fy) -> [Fy], Demux1/1  "Fy"
  Demux1/1 -> Vector Concatenate5/2
  Reshape6/1 -> Omega/1
  Wheel/1 -> Bus Selector7/1
  Vector Concatenate5/1 -> FrntAxlF/1
  Wheel to Body Transform/1(Fx) -> Demux/1, [Fx]  "Fx"
  Math Function/1 -> Wheel to Body Transform/1(Forces)
  Demux/1 -> Vector Concatenate5/1
  Demux1/2 -> Vector Concatenate6/2
  Demux/2 -> Vector Concatenate6/1
  Vector Concatenate6/1 -> MiddleAxlF/1
  Vector Concatenate8/1 -> Math Function/1
  Bus Selector7/2 -> Subsystem/1(<Fx>)  "<Fx>"
  Bus Selector7/3 -> Subsystem/2(<Fy>)  "<Fy>"
  Fz/1 -> Subsystem/3(Fz)
  Subsystem/1(FxTotal) -> Dead Zone2/1
  Subsystem/2(FyTotal) -> Dead Zone3/1
  Subsystem/3(FzTotal) -> Vector Concatenate8/3
  Dead Zone2/1 -> Vector Concatenate8/1
  Dead Zone3/1 -> Vector Concatenate8/2

== system TractorTrailer6DOF/Three-Axle Trailer/Wheels and Tires/Wheels and Tires/Tires ==
  "DriveTorque " : Inport
  "Brake Pressure " : Inport  Port=2
  "r " : Inport  Port=3
  "Vx " : Inport  Port=4
  "Vy " : Inport  Port=5
  "Camber " : Inport  Port=6
  "Press " : Inport  Port=7
  "lambda " : Inport  Port=8
  "Gnd " : Inport  Port=9
  "FzSusp " : Inport  Port=10
  Fiala Tires : Subsystem  VariantControl=1
  MF Tires : Subsystem  VariantControl=0
  " Wheels" : Outport  VectorParamsAs1DForOutWhenUnconnected=off

== system TractorTrailer6DOF/Three-Axle Trailer/Wheels and Tires/Wheels and Tires/Veh2Tire ==
  r : Inport
  Axle : Inport  Port=2
  Brake : Inport  Port=3
  VehVel : Inport  Port=4
  WheelSteer : Inport  Port=5
  WheelCamber : Inport  Port=6
  Demux4 : Demux  Outputs=6
  Gain4 : Gain  Gain=[1;-1;1;-1;1;-1]*0+1
  Mux1 : Mux  Inputs=6
  Reshape3 : Reshape
  Reshape4 : Reshape
  Unary Minus : UnaryMinus
  Wheel Angles : Subsystem
  Wheel to Body Transform : Subsystem
  T : Outport  Unit=N*m  VectorParamsAs1DForOutWhenUnconnected=off
  P : Outport  Port=2  Unit=Pa  PortDimensions=6  VectorParamsAs1DForOutWhenUnconnected=off
  psidot : Outport  Port=3  Unit=rad/s  VectorParamsAs1DForOutWhenUnconnected=off
  xdotAxle : Outport  Port=4  Unit=m/s  PortDimensions=6  VectorParamsAs1DForOutWhenUnconnected=off
  ydotAxle : Outport  Port=5  Unit=m/s  PortDimensions=6  VectorParamsAs1DForOutWhenUnconnected=off
  zdotAxle : Outport  Port=6  Unit=m/s  PortDimensions=6  VectorParamsAs1DForOutWhenUnconnected=off
  wires:
  Demux4/6 -> Mux1/6
  Demux4/5 -> Mux1/5
  Wheel Angles/1(Vehicle) -> Wheel to Body Transform/2(WheelAngles)
  Unary Minus/1 -> psidot/1
  WheelCamber/1 -> Wheel Angles/2(camber)
  Wheel to Body Transform/3(zdotWheel) -> zdotAxle/1  "Vz"
  VehVel/1 -> Wheel to Body Transform/1(VelVeh)
  Reshape4/1 -> Gain4/1
  Gain4/1 -> T/1
  Reshape3/1 -> Demux4/1
  Demux4/3 -> Mux1/3
  r/1 -> Unary Minus/1
  Mux1/1 -> P/1
  WheelSteer/1 -> Wheel Angles/1(steer)
  Wheel to Body Transform/2(ydotWheel) -> ydotAxle/1  "Vy"
  Demux4/2 -> Mux1/2
  Wheel to Body Transform/1(xdotWheel) -> xdotAxle/1  "Vx"
  Axle/1 -> Reshape4/1
  Demux4/4 -> Mux1/4
  Brake/1 -> Reshape3/1
  Demux4/1 -> Mux1/1

== system TractorTrailer6DOF/Three-Axle Trailer/Wheels and Tires/Wheels and Tires/scale factors with friction ==
  lamda_mu_x : Inport
  lamda_mu_y : Inport  Port=2
  0 : Constant  Value=[zeros(1,numWheels)]  VectorParams1D=off
  Reshape : Reshape  OutputDimensionality=Row vector (2-D)  OutputDimensions=[1,numWheels]
  Reshape1 : Reshape  OutputDimensionality=Row vector (2-D)  OutputDimensions=[1,numWheels]
  Signal Specification3 : SignalSpecification  Unit=1
  Vector Concatenate : Concatenate  NumInputs=5  Mode=Multidimensional array
  ones : Constant  Value=[ones(23,numWheels)]  VectorParams1D=off
  ones2 : Constant  Value=ones(1,numWheels)  VectorParams1D=off
  lambdas : Outport  Unit=1  VectorParamsAs1DForOutWhenUnconnected=off
  wires:
  lamda_mu_y/1 -> Reshape1/1
  lamda_mu_x/1 -> Reshape/1
  ones2/1 -> Vector Concatenate/1  "lambda_Fz0"
  Vector Concatenate/1 -> Signal Specification3/1
  ones/1 -> Vector Concatenate/5
  0/1 -> Vector Concatenate/4  "lamda_mu_V"
  Reshape1/1 -> Vector Concatenate/3
  Reshape/1 -> Vector Concatenate/2
  Signal Specification3/1 -> lambdas/1

== system TractorTrailer6DOF/Three-Axle Tractor/Wheels and Tires/Wheels and Tires/Tire2Veh/Routing ==
  <Mz> : Inport
  <Mx> : Inport  Port=2
  <My> : Inport  Port=3
  <Re> : Inport  Port=4
  <z> : Inport  Port=5
  <zdot> : Inport  Port=6
  <Kappa> : Inport  Port=7
  <Alpha> : Inport  Port=8
  Omega : Inport  Port=9
  Fx : Inport  Port=10
  Fy : Inport  Port=11
  Fz : Inport  Port=12
  Bus Creator : BusCreator  Inputs=12
  Reshape : Reshape  OutputDimensionality=Row vector (2-D)
  Reshape1 : Reshape  OutputDimensionality=Row vector (2-D)
  Unary Minus1 : UnaryMinus
  Unary Minus2 : UnaryMinus
  Out1 : Outport  VectorParamsAs1DForOutWhenUnconnected=off
  Out2 : Outport  Port=2  VectorParamsAs1DForOutWhenUnconnected=off
  Out3 : Outport  Port=3  VectorParamsAs1DForOutWhenUnconnected=off
  wires:
  <Re>/1 -> Bus Creator/8
  Unary Minus1/1 -> Reshape/1, Bus Creator/9  "z"
  Fz/1 -> Bus Creator/4
  <zdot>/1 -> Unary Minus2/1
  <Mz>/1 -> Bus Creator/7
  Unary Minus2/1 -> Reshape1/1, Bus Creator/10  "zdot"
  <z>/1 -> Unary Minus1/1
  Bus Creator/1 -> Out1/1
  Fy/1 -> Bus Creator/3
  Omega/1 -> Bus Creator/1  "Omega"
  Fx/1 -> Bus Creator/2
  Reshape1/1 -> Out3/1
  <Kappa>/1 -> Bus Creator/11
  Reshape/1 -> Out2/1
  <Mx>/1 -> Bus Creator/5
  <My>/1 -> Bus Creator/6
  <Alpha>/1 -> Bus Creator/12

== system TractorTrailer6DOF/Three-Axle Tractor/Wheels and Tires/Wheels and Tires/Tire2Veh/Subsystem1 ==
  Fin : Inport
  Demux : Demux  Outputs=6
  Gain10 : Gain  Gain=tractor.NumberOfWheelsPerMiddleAxle
  Gain11 : Gain  Gain=tractor.NumberOfWheelsPerMiddleAxle
  Gain12 : Gain  Gain=tractor.NumberOfWheelsPerRearAxle
  Gain13 : Gain  Gain=tractor.NumberOfWheelsPerRearAxle
  Gain14 : Gain  Gain=1/2
  Gain8 : Gain  Gain=tractor.NumberOfWheelsPerFrontAxle
  Gain9 : Gain  Gain=tractor.NumberOfWheelsPerFrontAxle
  Mux1 : Mux  Inputs=6
  Reshape : Reshape  OutputDimensionality=Column vector (2-D)
  Fout : Outport
  wires:
  Reshape/1 -> Fout/1
  Gain14/1 -> Reshape/1
  Demux/5 -> Gain12/1
  Demux/3 -> Gain10/1
  Demux/1 -> Gain8/1
  Demux/2 -> Gain9/1
  Gain12/1 -> Mux1/5
  Gain8/1 -> Mux1/1
  Gain9/1 -> Mux1/2
  Fin/1 -> Demux/1
  Gain10/1 -> Mux1/3
  Gain11/1 -> Mux1/4
  Demux/6 -> Gain13/1
  Demux/4 -> Gain11/1
  Gain13/1 -> Mux1/6
  Mux1/1 -> Gain14/1

== system TractorTrailer6DOF/Three-Axle Tractor/Wheels and Tires/Wheels and Tires/Tire2Veh/Subsystem2 ==
  Fin : Inport
  Demux : Demux  Outputs=6
  Gain10 : Gain  Gain=tractor.NumberOfWheelsPerMiddleAxle
  Gain11 : Gain  Gain=tractor.NumberOfWheelsPerMiddleAxle
  Gain12 : Gain  Gain=tractor.NumberOfWheelsPerRearAxle
  Gain13 : Gain  Gain=tractor.NumberOfWheelsPerRearAxle
  Gain14 : Gain  Gain=1/2
  Gain8 : Gain  Gain=tractor.NumberOfWheelsPerFrontAxle
  Gain9 : Gain  Gain=tractor.NumberOfWheelsPerFrontAxle
  Mux1 : Mux  Inputs=6
  Reshape : Reshape  OutputDimensionality=Column vector (2-D)
  Fout : Outport
  wires:
  Mux1/1 -> Gain14/1
  Gain13/1 -> Mux1/6
  Demux/4 -> Gain11/1
  Demux/6 -> Gain13/1
  Gain11/1 -> Mux1/4
  Gain10/1 -> Mux1/3
  Fin/1 -> Demux/1
  Gain9/1 -> Mux1/2
  Gain8/1 -> Mux1/1
  Gain12/1 -> Mux1/5
  Demux/2 -> Gain9/1
  Demux/1 -> Gain8/1
  Demux/3 -> Gain10/1
  Demux/5 -> Gain12/1
  Gain14/1 -> Reshape/1
  Reshape/1 -> Fout/1

== system TractorTrailer6DOF/Three-Axle Tractor/Wheels and Tires/Wheels and Tires/Tire2Veh/Subsystem3 ==
  Fin : Inport
  Demux : Demux  Outputs=6
  Gain10 : Gain  Gain=tractor.NumberOfWheelsPerMiddleAxle
  Gain11 : Gain  Gain=tractor.NumberOfWheelsPerMiddleAxle
  Gain12 : Gain  Gain=tractor.NumberOfWheelsPerRearAxle
  Gain13 : Gain  Gain=tractor.NumberOfWheelsPerRearAxle
  Gain14 : Gain  Gain=1/2
  Gain8 : Gain  Gain=tractor.NumberOfWheelsPerFrontAxle
  Gain9 : Gain  Gain=tractor.NumberOfWheelsPerFrontAxle
  Mux1 : Mux  Inputs=6
  Reshape : Reshape  OutputDimensionality=Column vector (2-D)
  Fout : Outport
  wires:
  Mux1/1 -> Gain14/1
  Gain13/1 -> Mux1/6
  Demux/4 -> Gain11/1
  Demux/6 -> Gain13/1
  Gain11/1 -> Mux1/4
  Gain10/1 -> Mux1/3
  Fin/1 -> Demux/1
  Gain9/1 -> Mux1/2
  Gain8/1 -> Mux1/1
  Gain12/1 -> Mux1/5
  Demux/2 -> Gain9/1
  Demux/1 -> Gain8/1
  Demux/3 -> Gain10/1
  Demux/5 -> Gain12/1
  Gain14/1 -> Reshape/1
  Reshape/1 -> Fout/1

== system TractorTrailer6DOF/Three-Axle Tractor/Wheels and Tires/Wheels and Tires/Tire2Veh/Wheel Angles ==
  Front : Inport
  Camber : Inport  Port=2
  Add1 : Sum
  Add2 : Sum
  Constant1 : Constant  Value=pi
  Constant2 : Constant  Value=[pi;0;pi;0;pi;0].*0+[0;pi;0;pi;0;pi].*.0
  Constant3 : Constant  Value=ones(1,6).*0
  Reshape : Reshape  OutputDimensionality=Row vector (2-D)
  Reshape1 : Reshape  OutputDimensionality=Row vector (2-D)
  Reshape2 : Reshape  OutputDimensionality=Row vector (2-D)
  Vector Concatenate3 : Concatenate  NumInputs=3  Mode=Multidimensional array
  Vehicle : Outport  VectorParamsAs1DForOutWhenUnconnected=off
  wires:
  Reshape/1 -> Vector Concatenate3/3
  Reshape2/1 -> Vector Concatenate3/2
  Vector Concatenate3/1 -> Vehicle/1
  Constant2/1 -> Add1/2
  Front/1 -> Add1/1
  Reshape1/1 -> Vector Concatenate3/1
  Constant3/1 -> Reshape2/1
  Add1/1 -> Reshape/1
  Camber/1 -> Add2/1
  Add2/1 -> Reshape1/1
  Constant1/1 -> Add2/2

== system TractorTrailer6DOF/Three-Axle Tractor/Wheels and Tires/Wheels and Tires/Tire2Veh/Wheel to Body Transform ==
  Forces : Inport  PortDimensions=[3,1]  Partition=on  PartitionDimension=2  PartitionWidth=1  PartitionOffset=0
  WheelAngles : Inport  Port=2  PortDimensions=[3,1]  Partition=on  PartitionDimension=2  PartitionWidth=1  PartitionOffset=0
  Demux1 : Demux  Outputs=3
  Divide1 : Product  Inputs=**  Multiplication=Matrix(*)
  For Each : ForEach  DisableCoverage=on
  Rotation Angles to Direction Cosine Matrix : sharedtransform/Rotation Angles to Direction Cosine Matrix  rotationOrder=ZYX  aMode=2
  Selector : Selector  InputPortWidth=3  IndexOptions=Index vector (dialog)  Indices=[3 2 1]  OutputSizes=1
  Fx : Outport  ConcatenationDimension=1  VectorParamsAs1DForOutWhenUnconnected=off
  Fy : Outport  Port=2  ConcatenationDimension=1  VectorParamsAs1DForOutWhenUnconnected=off
  Fz : Outport  Port=3  ConcatenationDimension=1  VectorParamsAs1DForOutWhenUnconnected=off
  wires:
  Divide1/1 -> Demux1/1
  Demux1/1 -> Fx/1
  Demux1/2 -> Fy/1
  Demux1/3 -> Fz/1
  Rotation Angles to Direction Cosine Matrix/1 -> Divide1/1
  Forces/1 -> Divide1/2
  WheelAngles/1 -> Selector/1
  Selector/1 -> Rotation Angles to Direction Cosine Matrix/1
